simulink model "b3"  (R2017b)
settings: Solver=FixedStepAuto  StartTime=0.0  StopTime=50  RelTol=1e-3
libraries: simulink x1
settings Model: Creator=taduc  LastModifiedBy=JusP

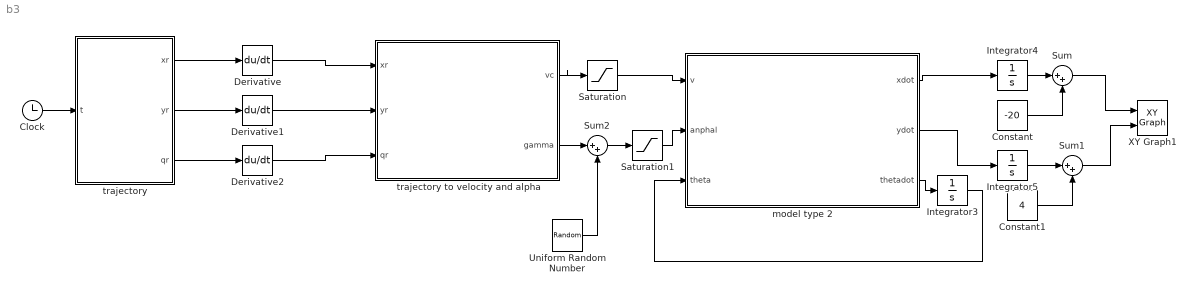
== system b3 ==
  Clock : Clock
  Constant : Constant  Value=-20
  Constant1 : Constant  Value=4
  Derivative : Derivative
  Derivative1 : Derivative
  Derivative2 : Derivative
  Integrator3 : Integrator
  Integrator4 : Integrator
  Integrator5 : Integrator
  Saturation : Saturate  UpperLimit=2  LowerLimit=-2
  Saturation1 : Saturate  UpperLimit=pi/4  LowerLimit=-pi/4
  Sum : Sum  Inputs=|++
  Sum1 : Sum  Inputs=|++
  Sum2 : Sum  Inputs=|++
  Uniform Random Number : UniformRandomNumber  Minimum=-5*pi/180  Maximum=5*pi/180  SampleTime=0.1
  XY Graph1 : simulink/Sinks/XY Graph  xmin=-20  xmax=5  ymin=-5  ymax=5  st=-1
  model type 2 : MATLAB Function  TreatAsAtomicUnit=on
  trajectory : MATLAB Function  TreatAsAtomicUnit=on
  trajectory to velocity and alpha : MATLAB Function  TreatAsAtomicUnit=on
  wires:
  model type 2/2(ydot) -> Integrator5/1
  Integrator3/1 -> model type 2/3(theta)
  model type 2/3(thetadot) -> Integrator3/1
  Clock/1 -> trajectory/1(t)
  trajectory/1(xr) -> Derivative/1
  Derivative/1 -> trajectory to velocity and alpha/1(xr)
  trajectory/2(yr) -> Derivative1/1
  Derivative1/1 -> trajectory to velocity and alpha/2(yr)
  trajectory/3(qr) -> Derivative2/1
  Derivative2/1 -> trajectory to velocity and alpha/3(qr)
  trajectory to velocity and alpha/1(vc) -> Saturation/1
  Saturation/1 -> model type 2/1(v)
  Saturation1/1 -> model type 2/2(anphal)
  model type 2/1(xdot) -> Integrator4/1
  Integrator4/1 -> Sum/1
  Constant/1 -> Sum/2
  Integrator5/1 -> Sum1/1
  Constant1/1 -> Sum1/2
  Sum/1 -> XY Graph1/1
  Sum1/1 -> XY Graph1/2
  Sum2/1 -> Saturation1/1
  trajectory to velocity and alpha/2(gamma) -> Sum2/1
  Uniform Random Number/1 -> Sum2/2

== matlab function b3/model type 2 ==
  data: v input; anphal input; theta input; xdot output; ydot output; thetadot output
function [xdot, ydot, thetadot]= tricycle_case_2a(v, anphal, theta)
g = 16;
d = sqrt(2.5+0.1*g);
xdot = v * cos(theta);
ydot = v * sin(theta);
thetadot = v/d*tan(anphal);

== matlab function b3/trajectory ==
  data: t input; xr output; yr output; qr output
function [xr,yr,qr] = trajectory(t)
if t < 20
    xr = -20 + t;
    yr = 4;
    qr = 0;
elseif t < 30
    xr = 4*sin(2*pi/20*(t-20));
    yr = 4*cos(2*pi/20*(t-20));
    qr = -2*pi/20*(t-20);
else
    xr = 30-t;
    yr = -4;
    qr = -pi;
end

== matlab function b3/trajectory to velocity and alpha ==
  data: xr input; vc output; yr input; qr input; gamma output
function [vc,gamma] = trajectory_to_velocity_and_gamma(xr,yr,qr)
g = 16;
d = sqrt(2.5+0.1*g);
vc = hypot(xr, yr);
gamma = atan2(d*qr, vc);
end
